simulink model "ex2"  (R2015a)
settings: Solver=ode3  StartTime=0.0  StopTime=0.05  FixedStep=2e-5  RelTol=1e-3
undefined symbols (not defined in the file or in its folder): gcbh, rcfiltgaincompat
libraries: commfilt2 x2, commrandsrc2 x1
settings Model: Creator=ctu  LastModifiedBy=ctu

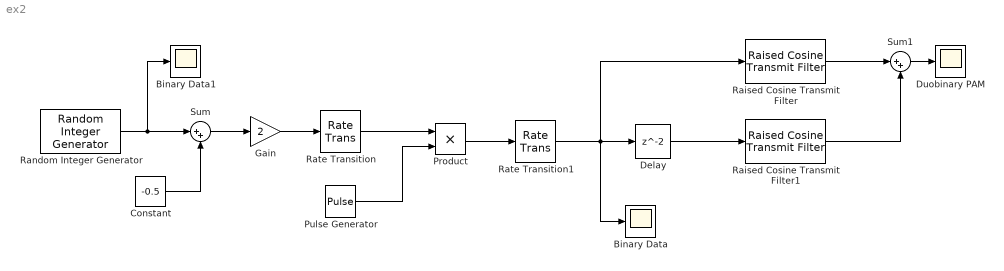
== system ex2 ==
  Binary Data : Scope
      settings: YMin=-1.5  YMax=1.5  SaveName=ScopeData2
  Binary Data1 : Scope
      settings: YMin=-0.5  YMax=1.5
  Constant : Constant  Value=-0.5
  Delay : Delay  InitialCondition=0  InputProcessing=Inherited
  Duobinary PAM : Scope
      settings: YMin=-15  YMax=15
  Gain : Gain  Gain=2
  Product : Product
  Pulse Generator : DiscretePulseGenerator  PulseType=Time based  Period=1e-3  PulseWidth=2
  Raised Cosine Transmit Filter : commfilt2/Raised Cosine Transmit Filter  filtType=Normal  filtSpan=8  currentFiltSpan=8  D=(8)/2  R=0  sampMode=Mute  saveAsFlag=0  N=50  framing=Allow multirate processing  InputProcessing=Inherited (this choice will be removed - see release notes)  checkGain=Normalized  filterGain=(5)*rcfiltgaincompat(gcbh)  checkCoeff=off  variableName=rcTxFilt  launchFVT=on  roundingMode=Floor  overflowMode=off
  Raised Cosine Transmit Filter1 : commfilt2/Raised Cosine Transmit Filter  filtType=Normal  filtSpan=8  currentFiltSpan=8  D=(8)/2  R=0  sampMode=Mute  saveAsFlag=0  N=50  framing=Allow multirate processing  InputProcessing=Inherited (this choice will be removed - see release notes)  checkGain=Normalized  filterGain=(5)*rcfiltgaincompat(gcbh)  checkCoeff=off  variableName=rcTxFilt1  launchFVT=on  roundingMode=Floor  overflowMode=off
  Random Integer Generator : commrandsrc2/Random Integer Generator  mul=2  seed=randseed  Ts=1e-3  frameBased=off  sampPerFrame=1  orient=off  outDataType=double
  Rate Transition : RateTransition  OutPortSampleTime=2e-5
  Rate Transition1 : RateTransition  OutPortSampleTime=1e-3
  Sum : Sum  Inputs=|++
  Sum1 : Sum  Inputs=|++
  wires:
  Random Integer Generator/1 -> Binary Data1/1, Sum/1
  Sum/1 -> Gain/1
  Constant/1 -> Sum/2
  Gain/1 -> Rate Transition/1
  Rate Transition/1 -> Product/1
  Pulse Generator/1 -> Product/2
  Product/1 -> Rate Transition1/1
  Sum1/1 -> Duobinary PAM/1
  Rate Transition1/1 -> Delay/1, Binary Data/1, Raised Cosine Transmit Filter/1
  Delay/1 -> Raised Cosine Transmit Filter1/1
  Raised Cosine Transmit Filter1/1 -> Sum1/2
  Raised Cosine Transmit Filter/1 -> Sum1/1
